simulink model "TST_HLSDem_SetPoint"  (R2016b)
settings: Solver=FixedStepDiscrete  StartTime=0.0  StopTime=simTime  FixedStep=sampleTime  RelTol=1e-3
values from neighbouring files (symbols this model uses):
  testCase = 1    [initTST_HLSDem_SetPoint_001.m]
libraries: simulink x5, UnitTest_Lib x3
settings Model: Creator=xuxingpei  LastModifiedBy=xuxingpei
settings DebuggingCC: SignalRangeChecking=error

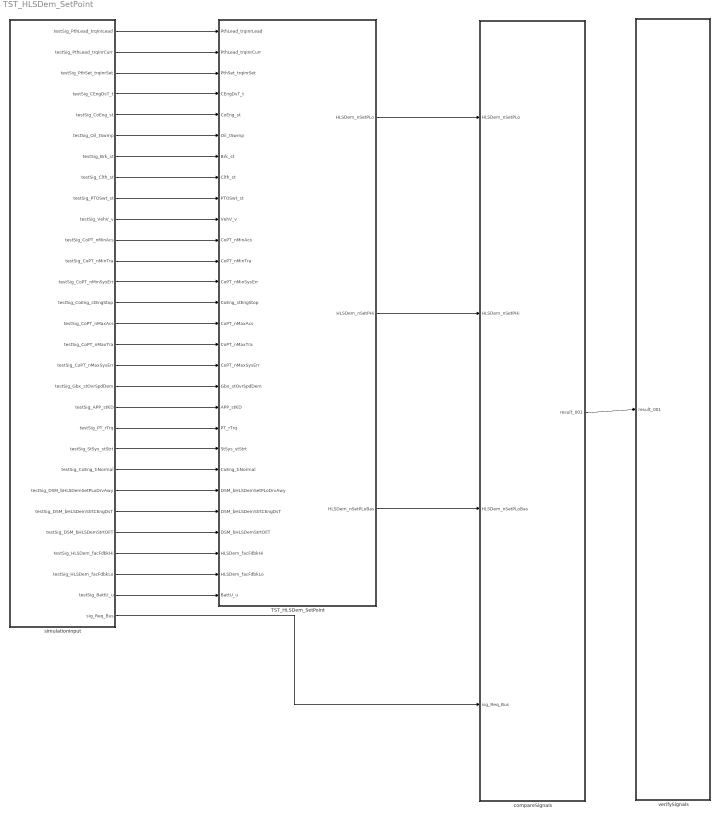
== system TST_HLSDem_SetPoint ==
  TST_HLSDem_SetPoint : Subsystem
  compareSignals : Subsystem
  simulationInput : Subsystem
  verifySignals : Subsystem
  wires:
  simulationInput/1(testSig_PthLead_trqInrLead) -> TST_HLSDem_SetPoint/1(PthLead_trqInrLead)
  simulationInput/2(testSig_PthLead_trqInrCurr) -> TST_HLSDem_SetPoint/2(PthLead_trqInrCurr)
  simulationInput/3(testSig_PthSet_trqInrSet) -> TST_HLSDem_SetPoint/3(PthSet_trqInrSet)
  simulationInput/4(testSig_CEngDsT_t) -> TST_HLSDem_SetPoint/4(CEngDsT_t)
  simulationInput/5(testSig_CoEng_st) -> TST_HLSDem_SetPoint/5(CoEng_st)
  simulationInput/6(testSig_Oil_tSwmp) -> TST_HLSDem_SetPoint/6(Oil_tSwmp)
  simulationInput/7(testSig_Brk_st) -> TST_HLSDem_SetPoint/7(Brk_st)
  simulationInput/8(testSig_Clth_st) -> TST_HLSDem_SetPoint/8(Clth_st)
  simulationInput/9(testSig_PTOSwt_st) -> TST_HLSDem_SetPoint/9(PTOSwt_st)
  simulationInput/10(testSig_VehV_v) -> TST_HLSDem_SetPoint/10(VehV_v)
  simulationInput/11(testSig_CoPT_nMinAcs) -> TST_HLSDem_SetPoint/11(CoPT_nMinAcs)
  simulationInput/12(testSig_CoPT_nMinTra) -> TST_HLSDem_SetPoint/12(CoPT_nMinTra)
  simulationInput/13(testSig_CoPT_nMinSysErr) -> TST_HLSDem_SetPoint/13(CoPT_nMinSysErr)
  simulationInput/14(testSig_CoEng_stEngStop) -> TST_HLSDem_SetPoint/14(CoEng_stEngStop)
  simulationInput/15(testSig_CoPT_nMaxAcs) -> TST_HLSDem_SetPoint/15(CoPT_nMaxAcs)
  simulationInput/16(testSig_CoPT_nMaxTra) -> TST_HLSDem_SetPoint/16(CoPT_nMaxTra)
  simulationInput/17(testSig_CoPT_nMaxSysErr) -> TST_HLSDem_SetPoint/17(CoPT_nMaxSysErr)
  simulationInput/18(testSig_Gbx_stOvrSpdDem) -> TST_HLSDem_SetPoint/18(Gbx_stOvrSpdDem)
  simulationInput/19(testSig_APP_stKD) -> TST_HLSDem_SetPoint/19(APP_stKD)
  simulationInput/20(testSig_PT_rTrq) -> TST_HLSDem_SetPoint/20(PT_rTrq)
  simulationInput/21(testSig_StSys_stStrt) -> TST_HLSDem_SetPoint/21(StSys_stStrt)
  simulationInput/22(testSig_CoEng_tiNormal) -> TST_HLSDem_SetPoint/22(CoEng_tiNormal)
  simulationInput/23(testSig_DSM_bHLSDemSetPLoDrvAwy) -> TST_HLSDem_SetPoint/23(DSM_bHLSDemSetPLoDrvAwy)
  simulationInput/24(testSig_DSM_bHLSDemStrtCEngDsT) -> TST_HLSDem_SetPoint/24(DSM_bHLSDemStrtCEngDsT)
  simulationInput/25(testSig_DSM_bHLSDemStrtOilT) -> TST_HLSDem_SetPoint/25(DSM_bHLSDemStrtOilT)
  simulationInput/26(testSig_HLSDem_facFdbkHi) -> TST_HLSDem_SetPoint/26(HLSDem_facFdbkHi)
  simulationInput/27(testSig_HLSDem_facFdbkLo) -> TST_HLSDem_SetPoint/27(HLSDem_facFdbkLo)
  simulationInput/28(testSig_BattU_u) -> TST_HLSDem_SetPoint/28(BattU_u)
  TST_HLSDem_SetPoint/1(HLSDem_nSetPLo) -> compareSignals/1(HLSDem_nSetPLo)
  TST_HLSDem_SetPoint/2(HLSDem_nSetPHi) -> compareSignals/2(HLSDem_nSetPHi)
  TST_HLSDem_SetPoint/3(HLSDem_nSetPLoBas) -> compareSignals/3(HLSDem_nSetPLoBas)
  simulationInput/29(sig_Req_Bus) -> compareSignals/4(sig_Req_Bus)
  compareSignals/1(result_001) -> verifySignals/1(result_001)

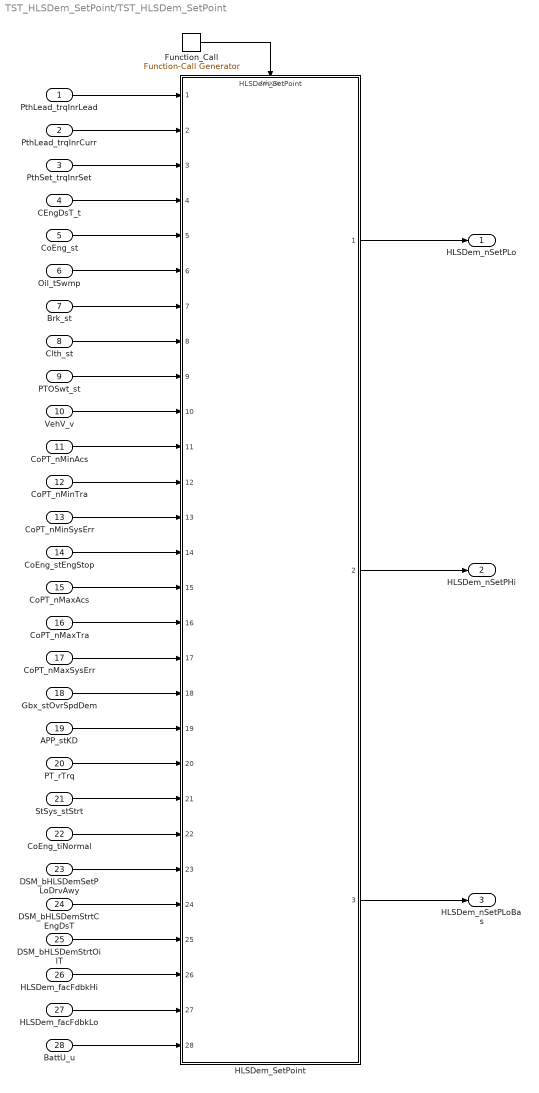
== system TST_HLSDem_SetPoint/TST_HLSDem_SetPoint ==
  PthLead_trqInrLead : Inport
  PthLead_trqInrCurr : Inport  Port=2
  PthSet_trqInrSet : Inport  Port=3
  CEngDsT_t : Inport  Port=4
  CoEng_st : Inport  Port=5
  Oil_tSwmp : Inport  Port=6
  Brk_st : Inport  Port=7
  Clth_st : Inport  Port=8
  PTOSwt_st : Inport  Port=9
  VehV_v : Inport  Port=10
  CoPT_nMinAcs : Inport  Port=11
  CoPT_nMinTra : Inport  Port=12
  CoPT_nMinSysErr : Inport  Port=13
  CoEng_stEngStop : Inport  Port=14
  CoPT_nMaxAcs : Inport  Port=15
  CoPT_nMaxTra : Inport  Port=16
  CoPT_nMaxSysErr : Inport  Port=17
  Gbx_stOvrSpdDem : Inport  Port=18
  APP_stKD : Inport  Port=19
  PT_rTrq : Inport  Port=20
  StSys_stStrt : Inport  Port=21
  CoEng_tiNormal : Inport  Port=22
  DSM_bHLSDemSetPLoDrvAwy : Inport  Port=23
  DSM_bHLSDemStrtCEngDsT : Inport  Port=24
  DSM_bHLSDemStrtOilT : Inport  Port=25
  HLSDem_facFdbkHi : Inport  Port=26
  HLSDem_facFdbkLo : Inport  Port=27
  BattU_u : Inport  Port=28
  Function_Call : simulink/Ports & Subsystems/Function-Call Generator  sample_time=sampleTime  numberOfIterations=1
  HLSDem_SetPoint : ModelReference  ModelNameDialog=HLSDem_SetPoint  SimulationMode=Normal  ModelReferenceVersion=1.107  TriggerPortName=function  TriggerPortTriggerType=function-call  TriggerPortStatesWhenEnabling=held
  HLSDem_nSetPLo : Outport
  HLSDem_nSetPHi : Outport  Port=2
  HLSDem_nSetPLoBas : Outport  Port=3
  wires:
  Function_Call/1 -> HLSDem_SetPoint/Trigger
  PthLead_trqInrLead/1 -> HLSDem_SetPoint/1
  PthLead_trqInrCurr/1 -> HLSDem_SetPoint/2
  PthSet_trqInrSet/1 -> HLSDem_SetPoint/3
  CEngDsT_t/1 -> HLSDem_SetPoint/4
  CoEng_st/1 -> HLSDem_SetPoint/5
  Oil_tSwmp/1 -> HLSDem_SetPoint/6
  Brk_st/1 -> HLSDem_SetPoint/7
  Clth_st/1 -> HLSDem_SetPoint/8
  PTOSwt_st/1 -> HLSDem_SetPoint/9
  VehV_v/1 -> HLSDem_SetPoint/10
  CoPT_nMinAcs/1 -> HLSDem_SetPoint/11
  CoPT_nMinTra/1 -> HLSDem_SetPoint/12
  CoPT_nMinSysErr/1 -> HLSDem_SetPoint/13
  CoEng_stEngStop/1 -> HLSDem_SetPoint/14
  CoPT_nMaxAcs/1 -> HLSDem_SetPoint/15
  CoPT_nMaxTra/1 -> HLSDem_SetPoint/16
  CoPT_nMaxSysErr/1 -> HLSDem_SetPoint/17
  Gbx_stOvrSpdDem/1 -> HLSDem_SetPoint/18
  APP_stKD/1 -> HLSDem_SetPoint/19
  PT_rTrq/1 -> HLSDem_SetPoint/20
  StSys_stStrt/1 -> HLSDem_SetPoint/21
  CoEng_tiNormal/1 -> HLSDem_SetPoint/22
  DSM_bHLSDemSetPLoDrvAwy/1 -> HLSDem_SetPoint/23
  DSM_bHLSDemStrtCEngDsT/1 -> HLSDem_SetPoint/24
  DSM_bHLSDemStrtOilT/1 -> HLSDem_SetPoint/25
  HLSDem_facFdbkHi/1 -> HLSDem_SetPoint/26
  HLSDem_facFdbkLo/1 -> HLSDem_SetPoint/27
  BattU_u/1 -> HLSDem_SetPoint/28
  HLSDem_SetPoint/1 -> HLSDem_nSetPLo/1
  HLSDem_SetPoint/2 -> HLSDem_nSetPHi/1
  HLSDem_SetPoint/3 -> HLSDem_nSetPLoBas/1

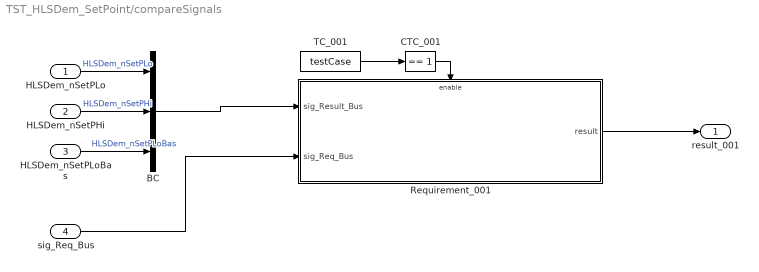
== system TST_HLSDem_SetPoint/compareSignals ==
  HLSDem_nSetPLo : Inport
  HLSDem_nSetPHi : Inport  Port=2
  HLSDem_nSetPLoBas : Inport  Port=3
  sig_Req_Bus : Inport  Port=4
  BC : BusCreator  Inputs=3
  CTC_001 : simulink/Logic and Bit Operations/Compare To Constant  relop===  const=1  OutDataTypeStr=boolean
  Requirement_001 : Subsystem
  TC_001 : Constant  Value=testCase
  result_001 : Outport
  wires:
  HLSDem_nSetPLo/1 -> BC/1  "HLSDem_nSetPLo"
  HLSDem_nSetPHi/1 -> BC/2  "HLSDem_nSetPHi"
  HLSDem_nSetPLoBas/1 -> BC/3  "HLSDem_nSetPLoBas"
  TC_001/1 -> CTC_001/1
  CTC_001/1 -> Requirement_001/Enable
  sig_Req_Bus/1 -> Requirement_001/2(sig_Req_Bus)
  BC/1 -> Requirement_001/1(sig_Result_Bus)
  Requirement_001/1(result) -> result_001/1

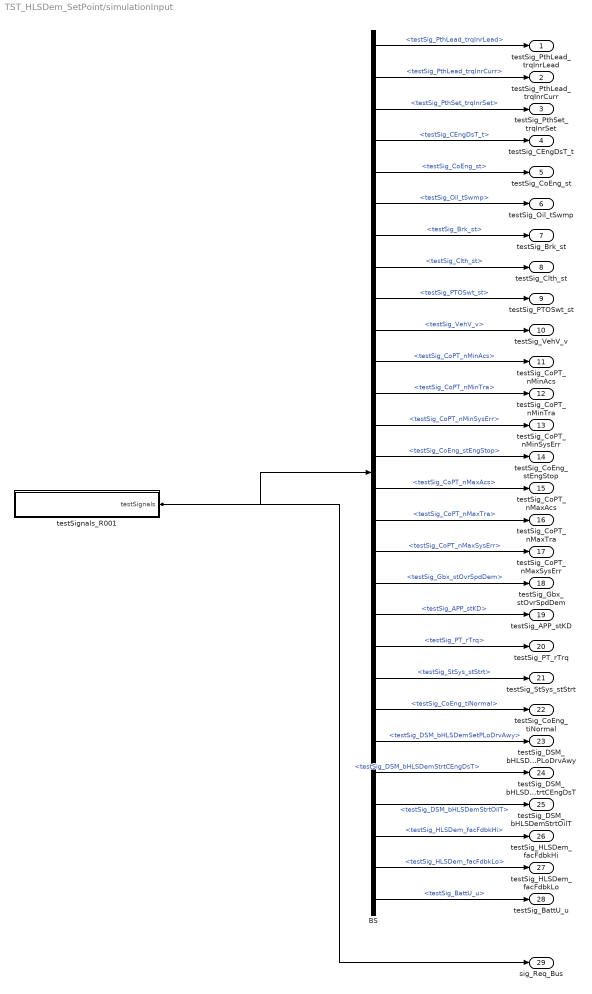
== system TST_HLSDem_SetPoint/simulationInput ==
  BS : BusSelector  OutputSignals=testSig_PthLead_trqInrLead,testSig_PthLead_trqInrCurr,testSig_PthSet_trqInrSet,testSig_CEngDsT_t,testSig_CoEng_st,testSig_Oil_tSwmp,testSig_Brk_st,testSig_Clth_st,testSig_PTOSwt_st,testSig_VehV_v,testSig_CoPT_nMinAcs,testSig_CoPT_nMinTra,testSig_CoPT_nMinSysErr,testSig_CoEng_stEngStop,testSig_CoPT_nMaxAcs,testSig_CoPT_nMaxTra,testSig_CoPT_nMaxSysErr,testSig_Gbx_stOvrSpdDem,testSig_APP_stKD,testSig_PT_rTrq,testSig_StSys_stStrt,testSig_CoEng_tiNormal,testSig_DSM_bHLSDemSetPLoDrvAwy,testSig_DSM_bHLSDemStrtCEngDsT,testSig_DSM_bHLSDemStrtOilT,testSig_HLSDem_facFdbkHi,testSig_HLSDem_facFdbkLo,testSig_BattU_u
  testSignals_R001 : Subsystem
  testSig_PthLead_trqInrLead : Outport
  testSig_PthLead_trqInrCurr : Outport  Port=2
  testSig_PthSet_trqInrSet : Outport  Port=3
  testSig_CEngDsT_t : Outport  Port=4
  testSig_CoEng_st : Outport  Port=5
  testSig_Oil_tSwmp : Outport  Port=6
  testSig_Brk_st : Outport  Port=7
  testSig_Clth_st : Outport  Port=8
  testSig_PTOSwt_st : Outport  Port=9
  testSig_VehV_v : Outport  Port=10
  testSig_CoPT_nMinAcs : Outport  Port=11
  testSig_CoPT_nMinTra : Outport  Port=12
  testSig_CoPT_nMinSysErr : Outport  Port=13
  testSig_CoEng_stEngStop : Outport  Port=14
  testSig_CoPT_nMaxAcs : Outport  Port=15
  testSig_CoPT_nMaxTra : Outport  Port=16
  testSig_CoPT_nMaxSysErr : Outport  Port=17
  testSig_Gbx_stOvrSpdDem : Outport  Port=18
  testSig_APP_stKD : Outport  Port=19
  testSig_PT_rTrq : Outport  Port=20
  testSig_StSys_stStrt : Outport  Port=21
  testSig_CoEng_tiNormal : Outport  Port=22
  testSig_DSM_bHLSDemSetPLoDrvAwy : Outport  Port=23
  testSig_DSM_bHLSDemStrtCEngDsT : Outport  Port=24
  testSig_DSM_bHLSDemStrtOilT : Outport  Port=25
  testSig_HLSDem_facFdbkHi : Outport  Port=26
  testSig_HLSDem_facFdbkLo : Outport  Port=27
  testSig_BattU_u : Outport  Port=28
  sig_Req_Bus : Outport  Port=29
  wires:
  BS/1 -> testSig_PthLead_trqInrLead/1  "<testSig_PthLead_trqInrLead>"
  BS/2 -> testSig_PthLead_trqInrCurr/1  "<testSig_PthLead_trqInrCurr>"
  BS/3 -> testSig_PthSet_trqInrSet/1  "<testSig_PthSet_trqInrSet>"
  BS/4 -> testSig_CEngDsT_t/1  "<testSig_CEngDsT_t>"
  BS/5 -> testSig_CoEng_st/1  "<testSig_CoEng_st>"
  BS/6 -> testSig_Oil_tSwmp/1  "<testSig_Oil_tSwmp>"
  BS/7 -> testSig_Brk_st/1  "<testSig_Brk_st>"
  BS/8 -> testSig_Clth_st/1  "<testSig_Clth_st>"
  BS/9 -> testSig_PTOSwt_st/1  "<testSig_PTOSwt_st>"
  BS/10 -> testSig_VehV_v/1  "<testSig_VehV_v>"
  BS/11 -> testSig_CoPT_nMinAcs/1  "<testSig_CoPT_nMinAcs>"
  BS/12 -> testSig_CoPT_nMinTra/1  "<testSig_CoPT_nMinTra>"
  BS/13 -> testSig_CoPT_nMinSysErr/1  "<testSig_CoPT_nMinSysErr>"
  BS/14 -> testSig_CoEng_stEngStop/1  "<testSig_CoEng_stEngStop>"
  BS/15 -> testSig_CoPT_nMaxAcs/1  "<testSig_CoPT_nMaxAcs>"
  BS/16 -> testSig_CoPT_nMaxTra/1  "<testSig_CoPT_nMaxTra>"
  BS/17 -> testSig_CoPT_nMaxSysErr/1  "<testSig_CoPT_nMaxSysErr>"
  BS/18 -> testSig_Gbx_stOvrSpdDem/1  "<testSig_Gbx_stOvrSpdDem>"
  BS/19 -> testSig_APP_stKD/1  "<testSig_APP_stKD>"
  BS/20 -> testSig_PT_rTrq/1  "<testSig_PT_rTrq>"
  BS/21 -> testSig_StSys_stStrt/1  "<testSig_StSys_stStrt>"
  BS/22 -> testSig_CoEng_tiNormal/1  "<testSig_CoEng_tiNormal>"
  BS/23 -> testSig_DSM_bHLSDemSetPLoDrvAwy/1  "<testSig_DSM_bHLSDemSetPLoDrvAwy>"
  BS/24 -> testSig_DSM_bHLSDemStrtCEngDsT/1  "<testSig_DSM_bHLSDemStrtCEngDsT>"
  BS/25 -> testSig_DSM_bHLSDemStrtOilT/1  "<testSig_DSM_bHLSDemStrtOilT>"
  BS/26 -> testSig_HLSDem_facFdbkHi/1  "<testSig_HLSDem_facFdbkHi>"
  BS/27 -> testSig_HLSDem_facFdbkLo/1  "<testSig_HLSDem_facFdbkLo>"
  BS/28 -> testSig_BattU_u/1  "<testSig_BattU_u>"
  testSignals_R001/1(testSignals) -> BS/1, sig_Req_Bus/1

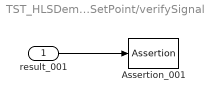
== system TST_HLSDem_SetPoint/verifySignals ==
  result_001 : Inport
  Assertion_001 : Assertion  Enabled=off
  wires:
  result_001/1 -> Assertion_001/1

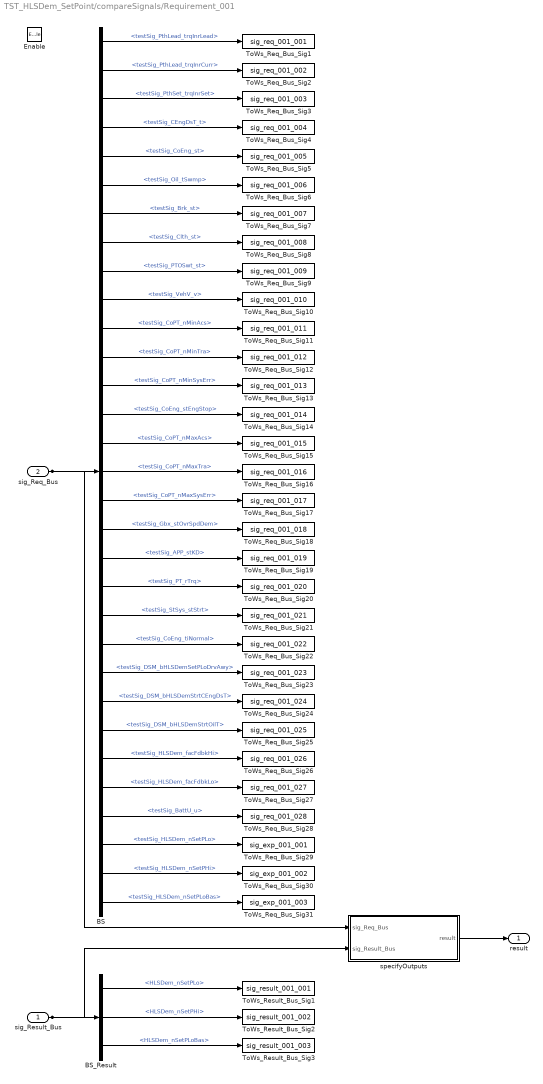
== system TST_HLSDem_SetPoint/compareSignals/Requirement_001 ==
  sig_Result_Bus : Inport
  sig_Req_Bus : Inport  Port=2
  Enable : EnablePort
  BS : BusSelector  OutputSignals=testSig_PthLead_trqInrLead,testSig_PthLead_trqInrCurr,testSig_PthSet_trqInrSet,testSig_CEngDsT_t,testSig_CoEng_st,testSig_Oil_tSwmp,testSig_Brk_st,testSig_Clth_st,testSig_PTOSwt_st,testSig_VehV_v,testSig_CoPT_nMinAcs,testSig_CoPT_nMinTra,testSig_CoPT_nMinSysErr,testSig_CoEng_stEngStop,testSig_CoPT_nMaxAcs,testSig_CoPT_nMaxTra,testSig_CoPT_nMaxSysErr,testSig_Gbx_stOvrSpdDem,testSig_APP_stKD,testSig_PT_rTrq,testSig_StSys_stStrt,testSig_CoEng_tiNormal,testSig_DSM_bHLSDemSetPLoDrvAwy,testSig_DSM_bHLSDemStrtCEngDsT,testSig_DSM_bHLSDemStrtOilT,testSig_HLSDem_facFdbkHi,testSig_HLSDem_facFdbkLo,testSig_BattU_u,testSig_HLSDem_nSetPLo,testSig_HLSDem_nSetPHi,testSig_HLSDem_nSetPLoBas
  BS_Result : BusSelector  OutputSignals=HLSDem_nSetPLo,HLSDem_nSetPHi,HLSDem_nSetPLoBas
  ToWs_Req_Bus_Sig1 : ToWorkspace  VariableName=sig_req_001_001  SaveFormat=Structure With Time
  ToWs_Req_Bus_Sig10 : ToWorkspace  VariableName=sig_req_001_010  SaveFormat=Structure With Time
  ToWs_Req_Bus_Sig11 : ToWorkspace  VariableName=sig_req_001_011  SaveFormat=Structure With Time
  ToWs_Req_Bus_Sig12 : ToWorkspace  VariableName=sig_req_001_012  SaveFormat=Structure With Time
  ToWs_Req_Bus_Sig13 : ToWorkspace  VariableName=sig_req_001_013  SaveFormat=Structure With Time
  ToWs_Req_Bus_Sig14 : ToWorkspace  VariableName=sig_req_001_014  SaveFormat=Structure With Time
  ToWs_Req_Bus_Sig15 : ToWorkspace  VariableName=sig_req_001_015  SaveFormat=Structure With Time
  ToWs_Req_Bus_Sig16 : ToWorkspace  VariableName=sig_req_001_016  SaveFormat=Structure With Time
  ToWs_Req_Bus_Sig17 : ToWorkspace  VariableName=sig_req_001_017  SaveFormat=Structure With Time
  ToWs_Req_Bus_Sig18 : ToWorkspace  VariableName=sig_req_001_018  SaveFormat=Structure With Time
  ToWs_Req_Bus_Sig19 : ToWorkspace  VariableName=sig_req_001_019  SaveFormat=Structure With Time
  ToWs_Req_Bus_Sig2 : ToWorkspace  VariableName=sig_req_001_002  SaveFormat=Structure With Time
  ToWs_Req_Bus_Sig20 : ToWorkspace  VariableName=sig_req_001_020  SaveFormat=Structure With Time
  ToWs_Req_Bus_Sig21 : ToWorkspace  VariableName=sig_req_001_021  SaveFormat=Structure With Time
  ToWs_Req_Bus_Sig22 : ToWorkspace  VariableName=sig_req_001_022  SaveFormat=Structure With Time
  ToWs_Req_Bus_Sig23 : ToWorkspace  VariableName=sig_req_001_023  SaveFormat=Structure With Time
  ToWs_Req_Bus_Sig24 : ToWorkspace  VariableName=sig_req_001_024  SaveFormat=Structure With Time
  ToWs_Req_Bus_Sig25 : ToWorkspace  VariableName=sig_req_001_025  SaveFormat=Structure With Time
  ToWs_Req_Bus_Sig26 : ToWorkspace  VariableName=sig_req_001_026  SaveFormat=Structure With Time
  ToWs_Req_Bus_Sig27 : ToWorkspace  VariableName=sig_req_001_027  SaveFormat=Structure With Time
  ToWs_Req_Bus_Sig28 : ToWorkspace  VariableName=sig_req_001_028  SaveFormat=Structure With Time
  ToWs_Req_Bus_Sig29 : ToWorkspace  VariableName=sig_exp_001_001  SaveFormat=Structure With Time
  ToWs_Req_Bus_Sig3 : ToWorkspace  VariableName=sig_req_001_003  SaveFormat=Structure With Time
  ToWs_Req_Bus_Sig30 : ToWorkspace  VariableName=sig_exp_001_002  SaveFormat=Structure With Time
  ToWs_Req_Bus_Sig31 : ToWorkspace  VariableName=sig_exp_001_003  SaveFormat=Structure With Time
  ToWs_Req_Bus_Sig4 : ToWorkspace  VariableName=sig_req_001_004  SaveFormat=Structure With Time
  ToWs_Req_Bus_Sig5 : ToWorkspace  VariableName=sig_req_001_005  SaveFormat=Structure With Time
  ToWs_Req_Bus_Sig6 : ToWorkspace  VariableName=sig_req_001_006  SaveFormat=Structure With Time
  ToWs_Req_Bus_Sig7 : ToWorkspace  VariableName=sig_req_001_007  SaveFormat=Structure With Time
  ToWs_Req_Bus_Sig8 : ToWorkspace  VariableName=sig_req_001_008  SaveFormat=Structure With Time
  ToWs_Req_Bus_Sig9 : ToWorkspace  VariableName=sig_req_001_009  SaveFormat=Structure With Time
  ToWs_Result_Bus_Sig1 : ToWorkspace  VariableName=sig_result_001_001  SaveFormat=Structure With Time
  ToWs_Result_Bus_Sig2 : ToWorkspace  VariableName=sig_result_001_002  SaveFormat=Structure With Time
  ToWs_Result_Bus_Sig3 : ToWorkspace  VariableName=sig_result_001_003  SaveFormat=Structure With Time
  specifyOutputs : Subsystem
  result : Outport
  wires:
  sig_Req_Bus/1 -> BS/1, specifyOutputs/1(sig_Req_Bus)
  BS/1 -> ToWs_Req_Bus_Sig1/1  "<testSig_PthLead_trqInrLead>"
  BS/2 -> ToWs_Req_Bus_Sig2/1  "<testSig_PthLead_trqInrCurr>"
  BS/3 -> ToWs_Req_Bus_Sig3/1  "<testSig_PthSet_trqInrSet>"
  BS/4 -> ToWs_Req_Bus_Sig4/1  "<testSig_CEngDsT_t>"
  BS/5 -> ToWs_Req_Bus_Sig5/1  "<testSig_CoEng_st>"
  BS/6 -> ToWs_Req_Bus_Sig6/1  "<testSig_Oil_tSwmp>"
  BS/7 -> ToWs_Req_Bus_Sig7/1  "<testSig_Brk_st>"
  BS/8 -> ToWs_Req_Bus_Sig8/1  "<testSig_Clth_st>"
  BS/9 -> ToWs_Req_Bus_Sig9/1  "<testSig_PTOSwt_st>"
  BS/10 -> ToWs_Req_Bus_Sig10/1  "<testSig_VehV_v>"
  BS/11 -> ToWs_Req_Bus_Sig11/1  "<testSig_CoPT_nMinAcs>"
  BS/12 -> ToWs_Req_Bus_Sig12/1  "<testSig_CoPT_nMinTra>"
  BS/13 -> ToWs_Req_Bus_Sig13/1  "<testSig_CoPT_nMinSysErr>"
  BS/14 -> ToWs_Req_Bus_Sig14/1  "<testSig_CoEng_stEngStop>"
  BS/15 -> ToWs_Req_Bus_Sig15/1  "<testSig_CoPT_nMaxAcs>"
  BS/16 -> ToWs_Req_Bus_Sig16/1  "<testSig_CoPT_nMaxTra>"
  BS/17 -> ToWs_Req_Bus_Sig17/1  "<testSig_CoPT_nMaxSysErr>"
  BS/18 -> ToWs_Req_Bus_Sig18/1  "<testSig_Gbx_stOvrSpdDem>"
  BS/19 -> ToWs_Req_Bus_Sig19/1  "<testSig_APP_stKD>"
  BS/20 -> ToWs_Req_Bus_Sig20/1  "<testSig_PT_rTrq>"
  BS/21 -> ToWs_Req_Bus_Sig21/1  "<testSig_StSys_stStrt>"
  BS/22 -> ToWs_Req_Bus_Sig22/1  "<testSig_CoEng_tiNormal>"
  BS/23 -> ToWs_Req_Bus_Sig23/1  "<testSig_DSM_bHLSDemSetPLoDrvAwy>"
  BS/24 -> ToWs_Req_Bus_Sig24/1  "<testSig_DSM_bHLSDemStrtCEngDsT>"
  BS/25 -> ToWs_Req_Bus_Sig25/1  "<testSig_DSM_bHLSDemStrtOilT>"
  BS/26 -> ToWs_Req_Bus_Sig26/1  "<testSig_HLSDem_facFdbkHi>"
  BS/27 -> ToWs_Req_Bus_Sig27/1  "<testSig_HLSDem_facFdbkLo>"
  BS/28 -> ToWs_Req_Bus_Sig28/1  "<testSig_BattU_u>"
  BS/29 -> ToWs_Req_Bus_Sig29/1  "<testSig_HLSDem_nSetPLo>"
  BS/30 -> ToWs_Req_Bus_Sig30/1  "<testSig_HLSDem_nSetPHi>"
  BS/31 -> ToWs_Req_Bus_Sig31/1  "<testSig_HLSDem_nSetPLoBas>"
  sig_Result_Bus/1 -> BS_Result/1, specifyOutputs/2(sig_Result_Bus)
  BS_Result/1 -> ToWs_Result_Bus_Sig1/1  "<HLSDem_nSetPLo>"
  BS_Result/2 -> ToWs_Result_Bus_Sig2/1  "<HLSDem_nSetPHi>"
  BS_Result/3 -> ToWs_Result_Bus_Sig3/1  "<HLSDem_nSetPLoBas>"
  specifyOutputs/1(result) -> result/1

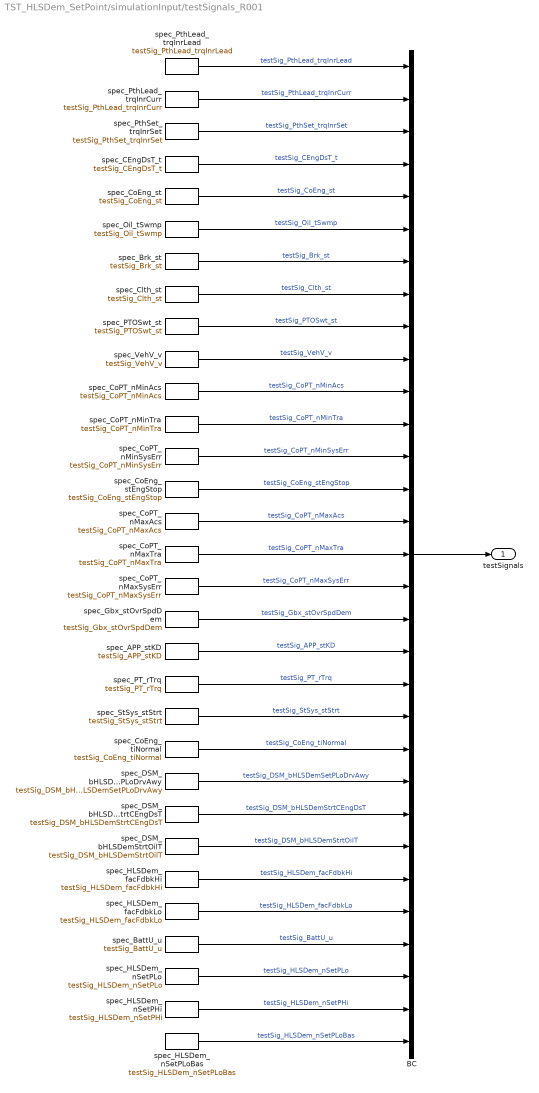
== system TST_HLSDem_SetPoint/simulationInput/testSignals_R001 ==
  BC : BusCreator  Inputs=31
  spec_APP_stKD : FromWorkspace  VariableName=testSig_APP_stKD  Interpolate=off  OutputAfterFinalValue=Holding final value
  spec_BattU_u : FromWorkspace  VariableName=testSig_BattU_u  Interpolate=off  OutputAfterFinalValue=Holding final value
  spec_Brk_st : FromWorkspace  VariableName=testSig_Brk_st  Interpolate=off  OutputAfterFinalValue=Holding final value
  spec_CEngDsT_t : FromWorkspace  VariableName=testSig_CEngDsT_t  Interpolate=off  OutputAfterFinalValue=Holding final value
  spec_Clth_st : FromWorkspace  VariableName=testSig_Clth_st  Interpolate=off  OutputAfterFinalValue=Holding final value
  spec_CoEng_st : FromWorkspace  VariableName=testSig_CoEng_st  Interpolate=off  OutputAfterFinalValue=Holding final value
  spec_CoEng_stEngStop : FromWorkspace  VariableName=testSig_CoEng_stEngStop  Interpolate=off  OutputAfterFinalValue=Holding final value
  spec_CoEng_tiNormal : FromWorkspace  VariableName=testSig_CoEng_tiNormal  Interpolate=off  OutputAfterFinalValue=Holding final value
  spec_CoPT_nMaxAcs : FromWorkspace  VariableName=testSig_CoPT_nMaxAcs  Interpolate=off  OutputAfterFinalValue=Holding final value
  spec_CoPT_nMaxSysErr : FromWorkspace  VariableName=testSig_CoPT_nMaxSysErr  Interpolate=off  OutputAfterFinalValue=Holding final value
  spec_CoPT_nMaxTra : FromWorkspace  VariableName=testSig_CoPT_nMaxTra  Interpolate=off  OutputAfterFinalValue=Holding final value
  spec_CoPT_nMinAcs : FromWorkspace  VariableName=testSig_CoPT_nMinAcs  Interpolate=off  OutputAfterFinalValue=Holding final value
  spec_CoPT_nMinSysErr : FromWorkspace  VariableName=testSig_CoPT_nMinSysErr  Interpolate=off  OutputAfterFinalValue=Holding final value
  spec_CoPT_nMinTra : FromWorkspace  VariableName=testSig_CoPT_nMinTra  Interpolate=off  OutputAfterFinalValue=Holding final value
  spec_DSM_bHLSDemSetPLoDrvAwy : FromWorkspace  VariableName=testSig_DSM_bHLSDemSetPLoDrvAwy  Interpolate=off  OutputAfterFinalValue=Holding final value
  spec_DSM_bHLSDemStrtCEngDsT : FromWorkspace  VariableName=testSig_DSM_bHLSDemStrtCEngDsT  Interpolate=off  OutputAfterFinalValue=Holding final value
  spec_DSM_bHLSDemStrtOilT : FromWorkspace  VariableName=testSig_DSM_bHLSDemStrtOilT  Interpolate=off  OutputAfterFinalValue=Holding final value
  spec_Gbx_stOvrSpdDem : FromWorkspace  VariableName=testSig_Gbx_stOvrSpdDem  Interpolate=off  OutputAfterFinalValue=Holding final value
  spec_HLSDem_facFdbkHi : FromWorkspace  VariableName=testSig_HLSDem_facFdbkHi  Interpolate=off  OutputAfterFinalValue=Holding final value
  spec_HLSDem_facFdbkLo : FromWorkspace  VariableName=testSig_HLSDem_facFdbkLo  Interpolate=off  OutputAfterFinalValue=Holding final value
  spec_HLSDem_nSetPHi : FromWorkspace  VariableName=testSig_HLSDem_nSetPHi  Interpolate=off  OutputAfterFinalValue=Holding final value
  spec_HLSDem_nSetPLo : FromWorkspace  VariableName=testSig_HLSDem_nSetPLo  Interpolate=off  OutputAfterFinalValue=Holding final value
  spec_HLSDem_nSetPLoBas : FromWorkspace  VariableName=testSig_HLSDem_nSetPLoBas  Interpolate=off  OutputAfterFinalValue=Holding final value
  spec_Oil_tSwmp : FromWorkspace  VariableName=testSig_Oil_tSwmp  Interpolate=off  OutputAfterFinalValue=Holding final value
  spec_PTOSwt_st : FromWorkspace  VariableName=testSig_PTOSwt_st  Interpolate=off  OutputAfterFinalValue=Holding final value
  spec_PT_rTrq : FromWorkspace  VariableName=testSig_PT_rTrq  Interpolate=off  OutputAfterFinalValue=Holding final value
  spec_PthLead_trqInrCurr : FromWorkspace  VariableName=testSig_PthLead_trqInrCurr  Interpolate=off  OutputAfterFinalValue=Holding final value
  spec_PthLead_trqInrLead : FromWorkspace  VariableName=testSig_PthLead_trqInrLead  Interpolate=off  OutputAfterFinalValue=Holding final value
  spec_PthSet_trqInrSet : FromWorkspace  VariableName=testSig_PthSet_trqInrSet  Interpolate=off  OutputAfterFinalValue=Holding final value
  spec_StSys_stStrt : FromWorkspace  VariableName=testSig_StSys_stStrt  Interpolate=off  OutputAfterFinalValue=Holding final value
  spec_VehV_v : FromWorkspace  VariableName=testSig_VehV_v  Interpolate=off  OutputAfterFinalValue=Holding final value
  testSignals : Outport
  wires:
  BC/1 -> testSignals/1
  spec_PthLead_trqInrLead/1 -> BC/1  "testSig_PthLead_trqInrLead"
  spec_PthLead_trqInrCurr/1 -> BC/2  "testSig_PthLead_trqInrCurr"
  spec_PthSet_trqInrSet/1 -> BC/3  "testSig_PthSet_trqInrSet"
  spec_CEngDsT_t/1 -> BC/4  "testSig_CEngDsT_t"
  spec_CoEng_st/1 -> BC/5  "testSig_CoEng_st"
  spec_Oil_tSwmp/1 -> BC/6  "testSig_Oil_tSwmp"
  spec_Brk_st/1 -> BC/7  "testSig_Brk_st"
  spec_Clth_st/1 -> BC/8  "testSig_Clth_st"
  spec_PTOSwt_st/1 -> BC/9  "testSig_PTOSwt_st"
  spec_VehV_v/1 -> BC/10  "testSig_VehV_v"
  spec_CoPT_nMinAcs/1 -> BC/11  "testSig_CoPT_nMinAcs"
  spec_CoPT_nMinTra/1 -> BC/12  "testSig_CoPT_nMinTra"
  spec_CoPT_nMinSysErr/1 -> BC/13  "testSig_CoPT_nMinSysErr"
  spec_CoEng_stEngStop/1 -> BC/14  "testSig_CoEng_stEngStop"
  spec_CoPT_nMaxAcs/1 -> BC/15  "testSig_CoPT_nMaxAcs"
  spec_CoPT_nMaxTra/1 -> BC/16  "testSig_CoPT_nMaxTra"
  spec_CoPT_nMaxSysErr/1 -> BC/17  "testSig_CoPT_nMaxSysErr"
  spec_Gbx_stOvrSpdDem/1 -> BC/18  "testSig_Gbx_stOvrSpdDem"
  spec_APP_stKD/1 -> BC/19  "testSig_APP_stKD"
  spec_PT_rTrq/1 -> BC/20  "testSig_PT_rTrq"
  spec_StSys_stStrt/1 -> BC/21  "testSig_StSys_stStrt"
  spec_CoEng_tiNormal/1 -> BC/22  "testSig_CoEng_tiNormal"
  spec_DSM_bHLSDemSetPLoDrvAwy/1 -> BC/23  "testSig_DSM_bHLSDemSetPLoDrvAwy"
  spec_DSM_bHLSDemStrtCEngDsT/1 -> BC/24  "testSig_DSM_bHLSDemStrtCEngDsT"
  spec_DSM_bHLSDemStrtOilT/1 -> BC/25  "testSig_DSM_bHLSDemStrtOilT"
  spec_HLSDem_facFdbkHi/1 -> BC/26  "testSig_HLSDem_facFdbkHi"
  spec_HLSDem_facFdbkLo/1 -> BC/27  "testSig_HLSDem_facFdbkLo"
  spec_BattU_u/1 -> BC/28  "testSig_BattU_u"
  spec_HLSDem_nSetPLo/1 -> BC/29  "testSig_HLSDem_nSetPLo"
  spec_HLSDem_nSetPHi/1 -> BC/30  "testSig_HLSDem_nSetPHi"
  spec_HLSDem_nSetPLoBas/1 -> BC/31  "testSig_HLSDem_nSetPLoBas"

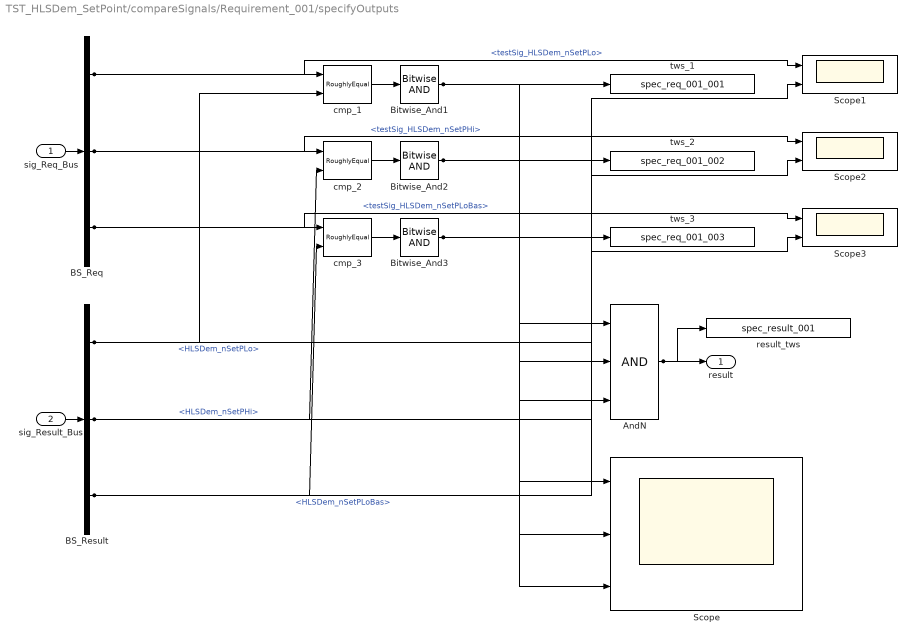
== system TST_HLSDem_SetPoint/compareSignals/Requirement_001/specifyOutputs ==
  sig_Req_Bus : Inport
  sig_Result_Bus : Inport  Port=2
  AndN : Logic  Inputs=3
  BS_Req : BusSelector  OutputSignals=testSig_HLSDem_nSetPLo,testSig_HLSDem_nSetPHi,testSig_HLSDem_nSetPLoBas
  BS_Result : BusSelector  OutputSignals=HLSDem_nSetPLo,HLSDem_nSetPHi,HLSDem_nSetPLoBas
  Bitwise_And1 : simulink/Logic and Bit Operations/Bitwise Operator  logicop=AND  UseBitMask=off  BitMask=bin2dec('11011001')  BitMaskRealWorld=Stored Integer
  Bitwise_And2 : simulink/Logic and Bit Operations/Bitwise Operator  logicop=AND  UseBitMask=off  BitMask=bin2dec('11011001')  BitMaskRealWorld=Stored Integer
  Bitwise_And3 : simulink/Logic and Bit Operations/Bitwise Operator  logicop=AND  UseBitMask=off  BitMask=bin2dec('11011001')  BitMaskRealWorld=Stored Integer
  Scope : Scope  NumInputPorts=3
  Scope1 : Scope  NumInputPorts=2
  Scope2 : Scope  NumInputPorts=2
  Scope3 : Scope  NumInputPorts=2
  cmp_1 : UnitTest_Lib/RoughlyEqual  slope=0.1
  cmp_2 : UnitTest_Lib/RoughlyEqual  slope=0.1
  cmp_3 : UnitTest_Lib/RoughlyEqual  slope=0.1
  result_tws : ToWorkspace  VariableName=spec_result_001
  tws_1 : ToWorkspace  VariableName=spec_req_001_001
  tws_2 : ToWorkspace  VariableName=spec_req_001_002
  tws_3 : ToWorkspace  VariableName=spec_req_001_003
  result : Outport
  wires:
  sig_Req_Bus/1 -> BS_Req/1
  sig_Result_Bus/1 -> BS_Result/1
  AndN/1 -> result/1, result_tws/1
  BS_Req/1 -> cmp_1/1, Scope1/1  "<testSig_HLSDem_nSetPLo>"
  BS_Result/1 -> cmp_1/2, Scope1/2  "<HLSDem_nSetPLo>"
  cmp_1/1 -> Bitwise_And1/1
  Bitwise_And1/1 -> tws_1/1, AndN/1, Scope/1
  BS_Req/2 -> cmp_2/1, Scope2/1  "<testSig_HLSDem_nSetPHi>"
  BS_Result/2 -> cmp_2/2, Scope2/2  "<HLSDem_nSetPHi>"
  cmp_2/1 -> Bitwise_And2/1
  Bitwise_And2/1 -> tws_2/1, AndN/2, Scope/2
  BS_Req/3 -> cmp_3/1, Scope3/1  "<testSig_HLSDem_nSetPLoBas>"
  BS_Result/3 -> cmp_3/2, Scope3/2  "<HLSDem_nSetPLoBas>"
  cmp_3/1 -> Bitwise_And3/1
  Bitwise_And3/1 -> tws_3/1, AndN/3, Scope/3
